simulink model "DC_Motor_Controller"  (R2021b)
settings: Solver=VariableStepAuto  StartTime=0.0  StopTime=20  RelTol=1e-3
libraries: PID_Controller_Library x1
settings Model: Creator=amr_y  LastModifiedBy=amr_y

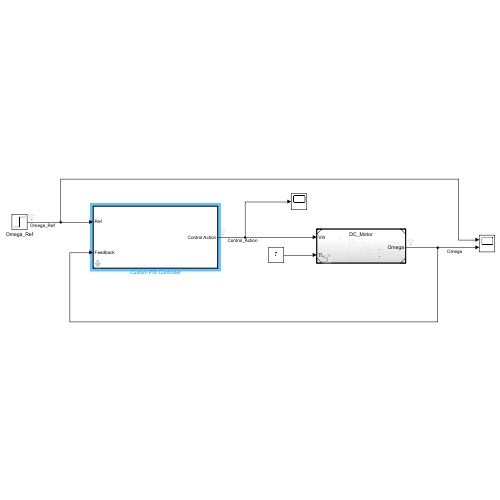
[thumbnail: Simulink's stored preview of the top-level diagram]
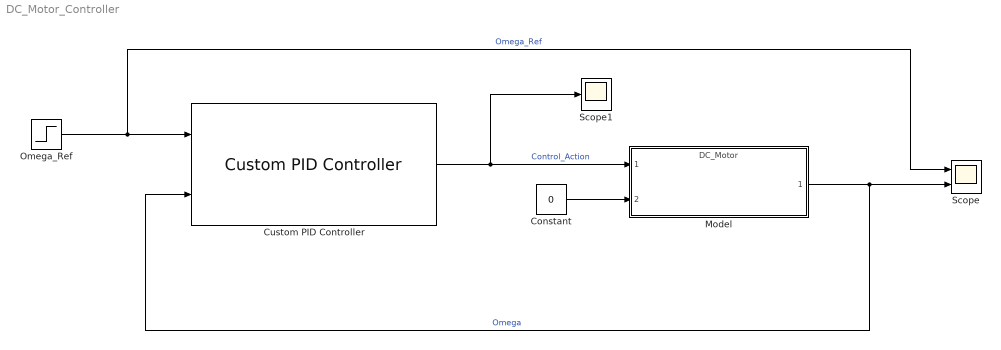
== system DC_Motor_Controller ==
  Constant : Constant  Value=0
  Custom PID Controller : PID_Controller_Library/Custom PID Controller  mask{Kp=1, Ki=1, Kd=0, Ic=0}
      mask prompts: Kp "Proportional"; Ki "Integeral"; Kd "differential"; Ic "Initial Condition"
      mask help:
      | Proportional is Kp gain
      | Integeral is Ki gain
      | Differential is Kd gain
  Model : ModelReference  ModelNameDialog=DC_Motor.slx  SimulationMode=Normal  ModelReferenceVersion=1.5
  Omega_Ref : Step  After=200  SampleTime=0
  Scope : Scope  NumInputPorts=2
  Scope1 : Scope
  wires:
  Custom PID Controller/1 -> Scope1/1, Model/1  "Control_Action"
  Omega_Ref/1 -> Scope/1, Custom PID Controller/1  "Omega_Ref"
  Model/1 -> Scope/2, Custom PID Controller/2  "Omega"
  Constant/1 -> Model/2
